simulink model "I_IOShxLTI_1"  (Simulink 5.0)
settings: Solver=ode45  StartTime=0.0  StopTime=20  RelTol=1e-3
libraries: cstblocks x2
settings Model: LastModifiedBy=User  BlockReductionOpt=off  BooleanDataType=off

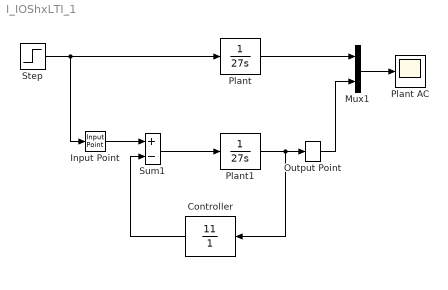
== system I_IOShxLTI_1 ==
  Controller : TransferFcn  Orientation=left  Numerator=[11]  Denominator=[0 1]
  Input Point : cstblocks/Input Point
  Mux1 : Mux  Inputs=2
  Output Point : cstblocks/Output Point
  Plant : TransferFcn  Denominator=[27 0]
  Plant AC : Scope
      settings: YMin=-5e+283  YMax=9e+284
  Plant1 : TransferFcn  Denominator=[27 0]
  Step : Step  Time=0.1  SampleTime=0
  Sum1 : Sum  Inputs=+-  SaturateOnIntegerOverflow=on  InputSameDT=on
  wires:
  Step/1 -> Plant/1, Input Point/1
  Plant/1 -> Mux1/1
  Sum1/1 -> Plant1/1
  Plant1/1 -> Controller/1, Output Point/1
  Mux1/1 -> Plant AC/1
  Controller/1 -> Sum1/2
  Input Point/1 -> Sum1/1
  Output Point/1 -> Mux1/2
